simulink model "impedance_match"  (R2024a)
settings: Solver=VariableStepAuto  StartTime=0.0  StopTime=10.0  RelTol=1e-3
undefined symbols (not defined in the file): Ts
libraries: fl_lib x16, nesl_utility x13, simulink x2, ee_lib x1
settings Model: Creator=gdudgeon  LastModifiedBy=sreinsel
settings DataIOCC: SaveOutput=off  DSMLogging=off  SaveTime=off  ReturnWorkspaceOutputs=off
settings OptimizationCC: ReuseModelBlockBuffer=off
settings DebuggingCC: UnconnectedInputMsg=warning  UnconnectedOutputMsg=warning  UnconnectedLineMsg=warning
settings ModelReferenceCC: EnableRefExpFcnMdlSchedulingChecks=on
settings RTWCC: GPUComputeCapability=3.5  DLArmComputeVersion=19.05

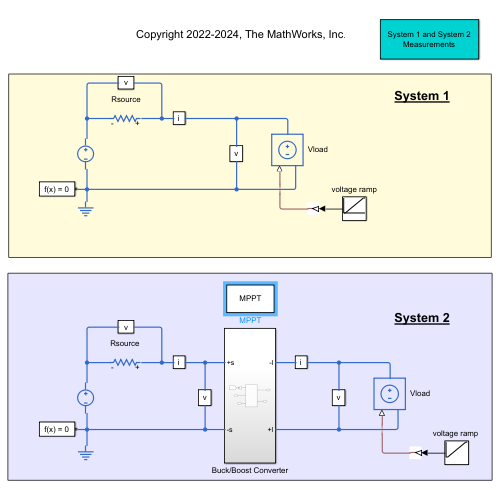
[thumbnail: Simulink's stored preview of the top-level diagram]
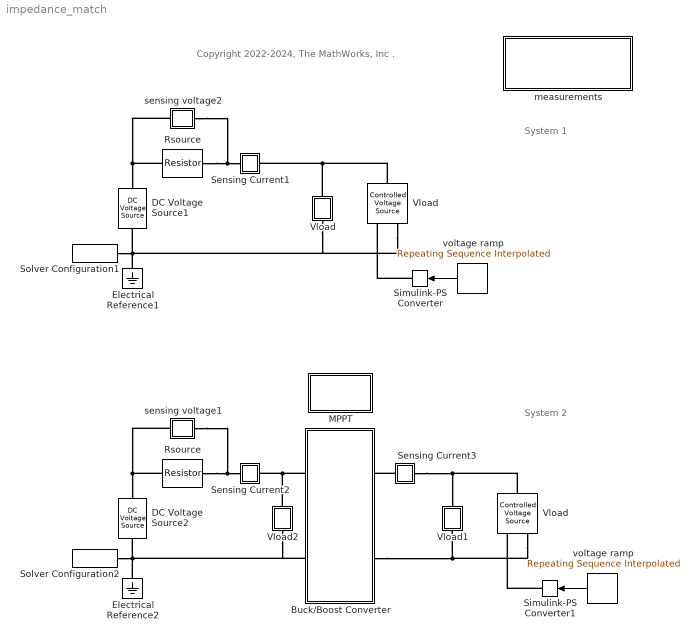
== system impedance_match ==
  note: Copyright 2022-2024, The MathWorks, Inc .
  note: System 2
  note: System 1
  Buck/Boost Converter : Subsystem
  DC Voltage Source1 : fl_lib/Electrical/Electrical Sources/DC Voltage Source  v0=200 V
  DC Voltage Source2 : fl_lib/Electrical/Electrical Sources/DC Voltage Source  v0=200 V
  Electrical Reference1 : fl_lib/Electrical/Electrical Elements/Electrical Reference
  Electrical Reference2 : fl_lib/Electrical/Electrical Elements/Electrical Reference
  MPPT : Subsystem
      mask Display: disp('MPPT')
  Rsource : fl_lib/Electrical/Electrical Elements/Resistor  R=100 Ohm  i_specify=off  i_priority=None  i=0 A  i_nominal_specify=off  i_nominal_value=1  i_nominal_unit=A  v_specify=off  v_priority=None  v=0 V  v_nominal_specify=off  v_nominal_value=1  v_nominal_unit=V
  "Rsource " : fl_lib/Electrical/Electrical Elements/Resistor  R=100 Ohm  i_specify=off  i_priority=None  i=0 A  i_nominal_specify=off  i_nominal_value=1  i_nominal_unit=A  v_specify=off  v_priority=None  v=0 V  v_nominal_specify=off  v_nominal_value=1  v_nominal_unit=V
  Sensing Current1 : Subsystem
      mask Display: disp('i')
  Sensing Current2 : Subsystem
      mask Display: disp('i')
  Sensing Current3 : Subsystem
      mask Display: disp('i')
  Simulink-PS Converter : nesl_utility/Simulink-PS Converter  PhysicalDomain=network_engine_domain  SubClassName=ps_input  LeftPortType=input  RightPortType=output  PseudoPeriodic=off  Frequencies=[]  NoiseDistribution=none  NoiseParameters=[]  Unit=1  AffineConversion=off  FilteringAndDerivatives=provide  SimscapeFilterOrder=1  InputFilterTimeConstant=0.001  UdotUserProvided=0
  Simulink-PS Converter1 : nesl_utility/Simulink-PS Converter  PhysicalDomain=network_engine_domain  SubClassName=ps_input  LeftPortType=input  RightPortType=output  PseudoPeriodic=off  Frequencies=[]  NoiseDistribution=none  NoiseParameters=[]  Unit=1  AffineConversion=off  FilteringAndDerivatives=provide  SimscapeFilterOrder=1  InputFilterTimeConstant=0.001  UdotUserProvided=0
  Solver Configuration1 : nesl_utility/Solver Configuration  PhysicalDomain=network_engine_domain  SubClassName=solver  LeftPortType=input  RightPortType=generic  Tones=[]  Harmonics=[]  SimulateNoise=off  Profile=off  UseLocalSampling=off  EnableSwitchedLinearOptims=on  FrequencyDomain=off  UseCCode=off  RelTol=0.001  AbsTol=1e-06  MinStep=1e-09  ToWorkspace=off  RevertToSquareIcSolve=off  NumHomotopyIterations=100  PhasorMode=off  PhasorModeNumHarmonics=1  ConsistencySolver=NEWTON_FTOL  IndexReductionMethod=DerivativeReplacement  DoDC=on  ResidualTolerance=1e-6  ConsistencyTolSource=GLOBAL  ConsistencyAbsTol=0.001  ConsistencyRelTol=0.001  ConsistencyTolFactor=0.001  UseLocalSolver=on  LocalSolverChoice=NE_BACKWARD_EULER_ADVANCER  ResolveIndetEquations=on  FunctionEvalNumThread=1  LocalSolverSampleTime=0.01  DoFixedCost=on  MaxNonlinIter=3  MaxModeIter=2  ComputeImpulses=off  ImpulseIterations=2  LinearAlgebra=auto  LinearAlgebraNumThread=0  EquationFormulation=NE_TIME_EF  DelaysMemoryBudget=1024  AutomaticFiltering=on  FilteringTimeConstant=0.001  PartitionStorageMethod=AS_NEEDED  PartitionMemoryBudget=1024  PartitionMethod=FAST  MultibodyUseLocalSolver=off  MultibodyLocalSolverChoice=ODE1  MultibodyLocalSolverSampleTime=0.001
  Solver Configuration2 : nesl_utility/Solver Configuration  PhysicalDomain=network_engine_domain  SubClassName=solver  LeftPortType=input  RightPortType=generic  Tones=[]  Harmonics=[]  SimulateNoise=off  Profile=off  UseLocalSampling=off  EnableSwitchedLinearOptims=on  FrequencyDomain=off  UseCCode=off  RelTol=0.001  AbsTol=1e-06  MinStep=1e-09  ToWorkspace=off  RevertToSquareIcSolve=off  NumHomotopyIterations=100  PhasorMode=off  PhasorModeNumHarmonics=1  ConsistencySolver=NEWTON_FTOL  IndexReductionMethod=DerivativeReplacement  DoDC=on  ResidualTolerance=1e-6  ConsistencyTolSource=GLOBAL  ConsistencyAbsTol=0.001  ConsistencyRelTol=0.001  ConsistencyTolFactor=0.001  UseLocalSolver=on  LocalSolverChoice=NE_BACKWARD_EULER_ADVANCER  ResolveIndetEquations=on  FunctionEvalNumThread=1  LocalSolverSampleTime=0.01  DoFixedCost=on  MaxNonlinIter=3  MaxModeIter=2  ComputeImpulses=off  ImpulseIterations=2  LinearAlgebra=auto  LinearAlgebraNumThread=0  EquationFormulation=NE_TIME_EF  DelaysMemoryBudget=1024  AutomaticFiltering=on  FilteringTimeConstant=0.001  PartitionStorageMethod=AS_NEEDED  PartitionMemoryBudget=1024  PartitionMethod=FAST  MultibodyUseLocalSolver=off  MultibodyLocalSolverChoice=ODE1  MultibodyLocalSolverSampleTime=0.001
  Vload : Subsystem
      mask Display: disp('v')
  "Vload " : fl_lib/Electrical/Electrical Sources/Controlled Voltage Source
  "Vload  " : fl_lib/Electrical/Electrical Sources/Controlled Voltage Source
  Vload1 : Subsystem
      mask Display: disp('v')
  Vload2 : Subsystem
      mask Display: disp('v')
  measurements : Subsystem
      mask Display: disp('System 1 and System 2\nMeasurements')
  sensing voltage1 : Subsystem
      mask Display: disp('v')
  sensing voltage2 : Subsystem
      mask Display: disp('v')
  voltage ramp : simulink/Sources/Repeating Sequence Interpolated  OutValues=[0 0 1 1]*200  TimeValues=[0 1 9 10]  LookUpMeth=Interpolation-Use End Values  tsamp=0.01  OutMin=[]  OutMax=[]  OutDataTypeStr=double  OutputDataTypeScalingMode=double  OutDataType=fixdt(0,8)  OutScaling=2^-10
  "voltage ramp " : simulink/Sources/Repeating Sequence Interpolated  OutValues=[0.1 0.1 1 1]*200  TimeValues=[0 1 9 10]  LookUpMeth=Interpolation-Use End Values  tsamp=0.01  OutMin=[]  OutMax=[]  OutDataTypeStr=double  OutputDataTypeScalingMode=double  OutDataType=fixdt(0,8)  OutScaling=2^-10
  wires:
  voltage ramp/1 -> Simulink-PS Converter/1
  "voltage ramp "/1 -> Simulink-PS Converter1/1
  connections:
  Electrical Reference1/LConn1 -- DC Voltage Source1/RConn1 -- Solver Configuration1/RConn1 -- "Vload "/RConn2 -- Vload/RConn1
  Vload/LConn1 -- "Vload "/LConn1 -- Sensing Current1/RConn1
  Rsource/LConn1 -- sensing voltage2/LConn1 -- Sensing Current1/LConn1
  Rsource/RConn1 -- sensing voltage2/RConn1 -- DC Voltage Source1/LConn1
  Simulink-PS Converter/RConn1 -- "Vload "/RConn1
  Solver Configuration2/RConn1 -- Buck/Boost Converter/LConn2 -- Vload2/RConn1 -- Electrical Reference2/LConn1 -- DC Voltage Source2/RConn1
  "Vload  "/LConn1 -- Sensing Current3/RConn1 -- Vload1/LConn1
  sensing voltage1/LConn1 -- "Rsource "/LConn1 -- Sensing Current2/LConn1
  "Rsource "/RConn1 -- DC Voltage Source2/LConn1 -- sensing voltage1/RConn1
  Simulink-PS Converter1/RConn1 -- "Vload  "/RConn1
  Vload2/LConn1 -- Sensing Current2/RConn1 -- Buck/Boost Converter/LConn1
  Buck/Boost Converter/RConn2 -- Vload1/RConn1 -- "Vload  "/RConn2
  Sensing Current3/LConn1 -- Buck/Boost Converter/RConn1

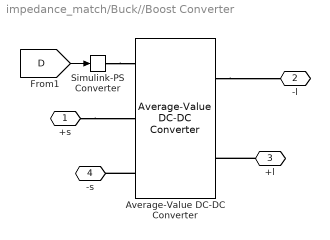
== system impedance_match/Buck//Boost Converter ==
  Average-Value DC-DC Converter : ee_lib/Semiconductors & Converters/Converters/Average-Value DC-DC Converter  control_option=ee.enum.converters.controlinput.dutycycle  converter_type=ee.enum.converters.dcdctype.boost  efficiency_option=ee.enum.converters.efficiency.constant  efficiency_fixed=100  i_vec=[0, 2, 5] A  efficiency_vec=[90, 95, 98]
      settings: InternalSimscapePortConfiguration="{\"Bottom\":[],\"Left\":[{\"id\":\"DutyCycle\",\"label\":\"DutyCycle\",\"type\":\"input\"},{\"id\":\"p1\",\"label\":\"1+\",\"type\":\"foundation.electrical.electrical\"},{\"id\":\"n1\",\"label\":\"1-\",\"type\":\"foundation.electrical.electrical\"}],\"Right\":[{\"id\":\"p2\",\"label\":\"2+\",\"type\":\"foundation.electrical.electrical\"},{\"id\":\"n2\",\"label\":\"2-\",\"type\":\"foundation.electrical.electrical\"}],\"Top\":[]}"
  Simulink-PS Converter : nesl_utility/Simulink-PS Converter  PhysicalDomain=network_engine_domain  SubClassName=ps_input  LeftPortType=input  RightPortType=output  PseudoPeriodic=off  Frequencies=[]  NoiseDistribution=none  NoiseParameters=[]  Unit=1  AffineConversion=off  FilteringAndDerivatives=provide  SimscapeFilterOrder=1  InputFilterTimeConstant=0.001  UdotUserProvided=0
  +s : PMIOPort  Side=Left
  -l : PMIOPort  Port=2  Side=Right
  +l : PMIOPort  Port=3  Side=Right
  -s : PMIOPort  Port=4  Side=Left
  wires:
  [D] -> Simulink-PS Converter/1
  connections:
  +s/RConn1 -- Average-Value DC-DC Converter/LConn2
  Average-Value DC-DC Converter/LConn3 -- -s/RConn1
  Simulink-PS Converter/RConn1 -- Average-Value DC-DC Converter/LConn1
  +l/RConn1 -- Average-Value DC-DC Converter/RConn2
  Average-Value DC-DC Converter/RConn1 -- -l/RConn1

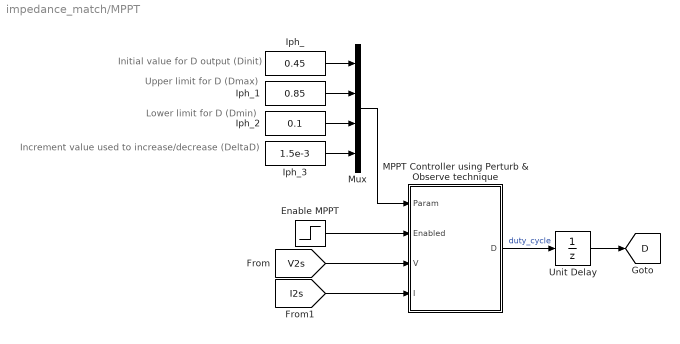
== system impedance_match/MPPT ==
  note: Lower limit for D (Dmin)
  note: Upper limit for D (Dmax)
  note: Increment value used to increase/decrease (DeltaD)
  note: Initial value for D output (Dinit)
  Enable MPPT : Step  Time=0.1  SampleTime=Ts
  Iph_ : Constant  Value=0.45
  Iph_1 : Constant  Value=0.85
  Iph_2 : Constant  Value=0.1
  Iph_3 : Constant  Value=1.5e-3
  "MPPT Controller using Perturb & Observe technique " : MATLAB Function  SystemSampleTime=Ts
  Mux : Mux
  Unit Delay : UnitDelay  InitialCondition=0.5  SampleTime=-1  HasFrameUpgradeWarning=on
  tag scope: D=global
  wires:
  Enable MPPT/1 -> "MPPT Controller using Perturb & Observe technique "/2(Enabled)
  Iph_3/1 -> Mux/4
  "MPPT Controller using Perturb & Observe technique "/1(D) -> Unit Delay/1  "duty_cycle"
  Iph_2/1 -> Mux/3
  Iph_/1 -> Mux/1
  Iph_1/1 -> Mux/2
  Mux/1 -> "MPPT Controller using Perturb & Observe technique "/1(Param)
  [V2s] -> "MPPT Controller using Perturb & Observe technique "/3(V)
  [I2s] -> "MPPT Controller using Perturb & Observe technique "/4(I)
  Unit Delay/1 -> [D]

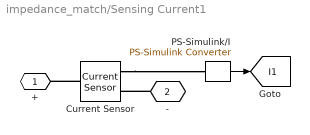
== system impedance_match/Sensing Current1 ==
  Current Sensor : fl_lib/Electrical/Electrical Sensors/Current Sensor
  PS-Simulink/I : nesl_utility/PS-Simulink Converter  PhysicalDomain=network_engine_domain  SubClassName=ps_output  LeftPortType=input  RightPortType=output  PseudoPeriodic=off  Frequencies=[]  VectorFormat=1-D array  Unit=1  AffineConversion=off
  + : PMIOPort  Side=Left
  - : PMIOPort  Port=2  Side=Right
  tag scope: I1=global
  wires:
  PS-Simulink/I/1 -> [I1]
  connections:
  Current Sensor/RConn1 -- PS-Simulink/I/LConn1
  Current Sensor/LConn1 -- +/RConn1
  -/RConn1 -- Current Sensor/RConn2

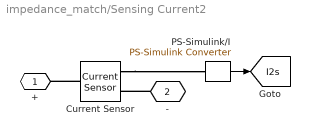
== system impedance_match/Sensing Current2 ==
  Current Sensor : fl_lib/Electrical/Electrical Sensors/Current Sensor
  PS-Simulink/I : nesl_utility/PS-Simulink Converter  PhysicalDomain=network_engine_domain  SubClassName=ps_output  LeftPortType=input  RightPortType=output  PseudoPeriodic=off  Frequencies=[]  VectorFormat=1-D array  Unit=1  AffineConversion=off
  + : PMIOPort  Side=Left
  - : PMIOPort  Port=2  Side=Right
  tag scope: I2s=global
  wires:
  PS-Simulink/I/1 -> [I2s]
  connections:
  -/RConn1 -- Current Sensor/RConn2
  Current Sensor/LConn1 -- +/RConn1
  Current Sensor/RConn1 -- PS-Simulink/I/LConn1

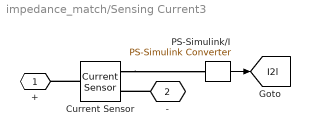
== system impedance_match/Sensing Current3 ==
  Current Sensor : fl_lib/Electrical/Electrical Sensors/Current Sensor
  PS-Simulink/I : nesl_utility/PS-Simulink Converter  PhysicalDomain=network_engine_domain  SubClassName=ps_output  LeftPortType=input  RightPortType=output  PseudoPeriodic=off  Frequencies=[]  VectorFormat=1-D array  Unit=1  AffineConversion=off
  + : PMIOPort  Side=Left
  - : PMIOPort  Port=2  Side=Right
  tag scope: I2l=global
  wires:
  PS-Simulink/I/1 -> [I2l]
  connections:
  Current Sensor/RConn1 -- PS-Simulink/I/LConn1
  Current Sensor/LConn1 -- +/RConn1
  -/RConn1 -- Current Sensor/RConn2

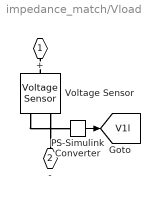
== system impedance_match/Vload ==
  PS-Simulink Converter : nesl_utility/PS-Simulink Converter  PhysicalDomain=network_engine_domain  SubClassName=ps_output  LeftPortType=input  RightPortType=output  PseudoPeriodic=off  Frequencies=[]  VectorFormat=1-D array  Unit=inherit  AffineConversion=off
  Voltage Sensor : fl_lib/Electrical/Electrical Sensors/Voltage Sensor
  + : PMIOPort  Side=Left
  - : PMIOPort  Port=2  Side=Right
  tag scope: V1l=global
  wires:
  PS-Simulink Converter/1 -> [V1l]
  connections:
  Voltage Sensor/RConn1 -- PS-Simulink Converter/LConn1
  Voltage Sensor/RConn2 -- -/RConn1
  Voltage Sensor/LConn1 -- +/RConn1

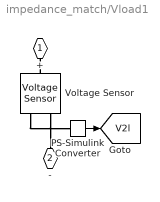
== system impedance_match/Vload1 ==
  PS-Simulink Converter : nesl_utility/PS-Simulink Converter  PhysicalDomain=network_engine_domain  SubClassName=ps_output  LeftPortType=input  RightPortType=output  PseudoPeriodic=off  Frequencies=[]  VectorFormat=1-D array  Unit=inherit  AffineConversion=off
  Voltage Sensor : fl_lib/Electrical/Electrical Sensors/Voltage Sensor
  + : PMIOPort  Side=Left
  - : PMIOPort  Port=2  Side=Right
  tag scope: V2l=global
  wires:
  PS-Simulink Converter/1 -> [V2l]
  connections:
  Voltage Sensor/LConn1 -- +/RConn1
  Voltage Sensor/RConn2 -- -/RConn1
  Voltage Sensor/RConn1 -- PS-Simulink Converter/LConn1

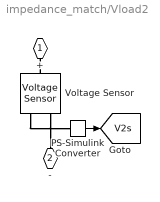
== system impedance_match/Vload2 ==
  PS-Simulink Converter : nesl_utility/PS-Simulink Converter  PhysicalDomain=network_engine_domain  SubClassName=ps_output  LeftPortType=input  RightPortType=output  PseudoPeriodic=off  Frequencies=[]  VectorFormat=1-D array  Unit=inherit  AffineConversion=off
  Voltage Sensor : fl_lib/Electrical/Electrical Sensors/Voltage Sensor
  + : PMIOPort  Side=Left
  - : PMIOPort  Port=2  Side=Right
  tag scope: V2s=global
  wires:
  PS-Simulink Converter/1 -> [V2s]
  connections:
  Voltage Sensor/RConn1 -- PS-Simulink Converter/LConn1
  Voltage Sensor/RConn2 -- -/RConn1
  Voltage Sensor/LConn1 -- +/RConn1

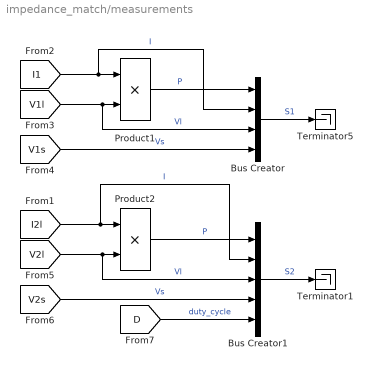
== system impedance_match/measurements ==
  Bus Creator : BusCreator  Inputs=4
  Bus Creator1 : BusCreator  Inputs=5
  Product1 : Product
  Product2 : Product
  Terminator1 : Terminator
  Terminator5 : Terminator
  wires:
  [V1l] -> Bus Creator/3, Product1/2  "Vl"
  [I1] -> Bus Creator/2, Product1/1  "I"
  [V1s] -> Bus Creator/4  "Vs"
  [I2l] -> Bus Creator1/2, Product2/1  "I"
  Product2/1 -> Bus Creator1/1  "P"
  [V2l] -> Bus Creator1/3, Product2/2  "Vl"
  [V2s] -> Bus Creator1/4  "Vs"
  Bus Creator/1 -> Terminator5/1  "S1"
  Product1/1 -> Bus Creator/1  "P"
  Bus Creator1/1 -> Terminator1/1  "S2"
  [D] -> Bus Creator1/5  "duty_cycle"

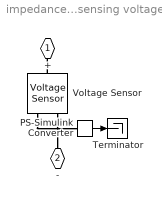
== system impedance_match/sensing voltage1 ==
  PS-Simulink Converter : nesl_utility/PS-Simulink Converter  PhysicalDomain=network_engine_domain  SubClassName=ps_output  LeftPortType=input  RightPortType=output  PseudoPeriodic=off  Frequencies=[]  VectorFormat=1-D array  Unit=inherit  AffineConversion=off
  Terminator : Terminator
  Voltage Sensor : fl_lib/Electrical/Electrical Sensors/Voltage Sensor
  + : PMIOPort  Side=Right
  - : PMIOPort  Port=2  Side=Left
  wires:
  PS-Simulink Converter/1 -> Terminator/1
  connections:
  Voltage Sensor/RConn1 -- PS-Simulink Converter/LConn1
  Voltage Sensor/RConn2 -- -/RConn1
  Voltage Sensor/LConn1 -- +/RConn1

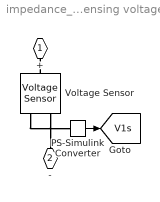
== system impedance_match/sensing voltage2 ==
  PS-Simulink Converter : nesl_utility/PS-Simulink Converter  PhysicalDomain=network_engine_domain  SubClassName=ps_output  LeftPortType=input  RightPortType=output  PseudoPeriodic=off  Frequencies=[]  VectorFormat=1-D array  Unit=inherit  AffineConversion=off
  Voltage Sensor : fl_lib/Electrical/Electrical Sensors/Voltage Sensor
  + : PMIOPort  Side=Right
  - : PMIOPort  Port=2  Side=Left
  tag scope: V1s=global
  wires:
  PS-Simulink Converter/1 -> [V1s]
  connections:
  Voltage Sensor/LConn1 -- +/RConn1
  Voltage Sensor/RConn2 -- -/RConn1
  Voltage Sensor/RConn1 -- PS-Simulink Converter/LConn1

== matlab function impedance_match/MPPT/MPPT Controller using Perturb & Observe technique  ==
  settings: updateMethod=DISCRETE  sampleTime=Ts
  data: Param input; Enabled input; V input; I input; D output
function D  = PandO(Param, Enabled, V, I)

% MPPT controller based on the Perturb & Observe algorithm.

% D output = Duty cycle of the boost converter (value between 0 and 1)
%
% Enabled input = 1 to enable the MPPT controller
% V input = PV array terminal voltage (V)
% I input = PV array current (A)
%
% Param input:
Dinit = Param(1);  %Initial value for D output
Dmax = Param(2);   %Maximum value for D
Dmin = Param(3);   %Minimum value for D
deltaD = Param(4); %Increment value used to increase/decrease the duty cycle D
% ( increasing D = decreasing Vref )
%  

persistent Vold Pold Dold;

dataType = 'double';

if isempty(Vold)
    Vold=0;
    Pold=0;
    Dold=Dinit;
end
P= V*I;
dV= V - Vold;
dP= P - Pold;

 if dP ~= 0 & Enabled ~=0
%     if dP>1e-9  & dP<-1e-9 & Enabled ~=0
    if dP < 0
        if dV < 0
            D = Dold - deltaD;
        else
            D = Dold + deltaD;
        end
    else
        if dV < 0
            D = Dold + deltaD;
        else
            D = Dold - deltaD;
        end    
    end
else D=Dold;
end

if D >= Dmax | D<= Dmin
    D=Dold;
end

Dold=D;
Vold=V;
Pold=P;
